simulink model "run_small_function_cov_bf"  (R2022b)
settings: Solver=VariableStepAuto  StartTime=0.0  StopTime=10.0  RelTol=1e-3
libraries: hdlsllib x39, ece1718_small_function x19, simulink x9
settings Model: SimulationMode=accelerator  Creator=kevin  LastModifiedBy=zishu wu

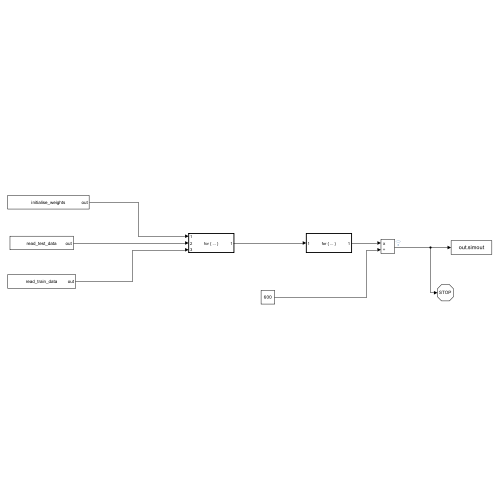
[thumbnail: Simulink's stored preview of the top-level diagram]
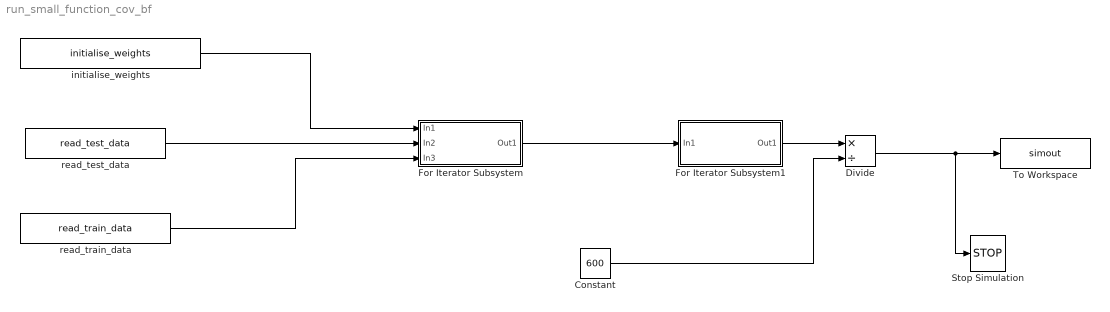
== system run_small_function_cov_bf ==
  Constant : Constant  Value=600
  Divide : Product  Inputs=*/  OutDataTypeStr=double
  For Iterator Subsystem : Subsystem  TreatAsAtomicUnit=on
  For Iterator Subsystem1 : Subsystem  TreatAsAtomicUnit=on
  Stop Simulation : Stop
  To Workspace : ToWorkspace  VariableName=simout  SaveFormat=Timeseries  SampleTime=-1
  initialise_weights : ece1718_small_function/initialise_weights  SampleTime=-1
  read_test_data : ece1718_small_function/read_test_data  SampleTime=-1
  read_train_data : ece1718_small_function/read_train_data  SampleTime=-1
  wires:
  For Iterator Subsystem/1(Out1) -> For Iterator Subsystem1/1(In1)
  read_test_data/1 -> For Iterator Subsystem/2(In2)
  read_train_data/1 -> For Iterator Subsystem/3(In3)
  For Iterator Subsystem1/1(Out1) -> Divide/1
  Constant/1 -> Divide/2
  Divide/1 -> Stop Simulation/1, To Workspace/1
  initialise_weights/1 -> For Iterator Subsystem/1(In1)

== system run_small_function_cov_bf/For Iterator Subsystem ==
  In1 : Inport
  In2 : Inport  Port=2
  In3 : Inport  Port=3
  For Iterator : ForIterator  ResetStates=reset  IterationLimit=1  IndexMode=Zero-based
  train_top : Subsystem  TreatAsAtomicUnit=on
  Out1 : Outport
  wires:
  In1/1 -> Out1/1
  For Iterator/1 -> train_top/1(In1)

== system run_small_function_cov_bf/For Iterator Subsystem1 ==
  In1 : Inport
  Delay : Delay  DelayLength=1  InitialCondition=0
  For Iterator : ForIterator  IterationLimit=600  IndexMode=Zero-based
  validate : ece1718_small_function/validate  SampleTime=-1
  Out1 : Outport
  wires:
  validate/1 -> Delay/1, Out1/1
  For Iterator/1 -> validate/1
  Delay/1 -> validate/2

== system run_small_function_cov_bf/For Iterator Subsystem/train_top ==
  In1 : Inport
  For Iterator : ForIterator  ResetStates=reset  IterationLimit=1  IndexMode=Zero-based
  batch : Subsystem
  Output : Outport
  wires:
  For Iterator/1 -> batch/1(Input)
  In1/1 -> Output/1

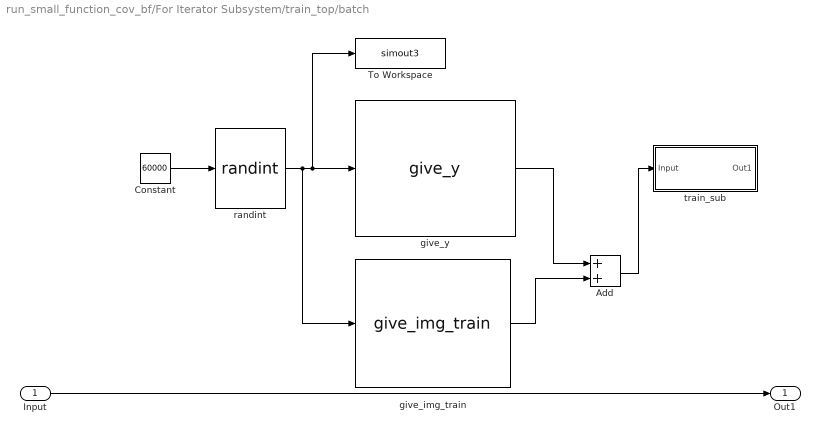
== system run_small_function_cov_bf/For Iterator Subsystem/train_top/batch ==
  Input : Inport
  Add : Sum
  Constant : Constant  Value=60000  OutDataTypeStr=int32
  To Workspace : ToWorkspace  VariableName=simout3  SaveFormat=Timeseries  SampleTime=-1
  give_img_train : ece1718_small_function/give_img_train  SampleTime=-1
  give_y : ece1718_small_function/give_y  SampleTime=-1
  randint : ece1718_small_function/randint  SampleTime=-1
  train_sub : Subsystem
      settings: LibrarySourceBlock=|
      | hdlsllib/Ports &
      | Subsystems/Subsystem
  Out1 : Outport
  wires:
  give_y/1 -> Add/1
  randint/1 -> give_img_train/1, To Workspace/1, give_y/1
  Constant/1 -> randint/1
  Input/1 -> Out1/1
  give_img_train/1 -> Add/2
  Add/1 -> train_sub/1(Input)

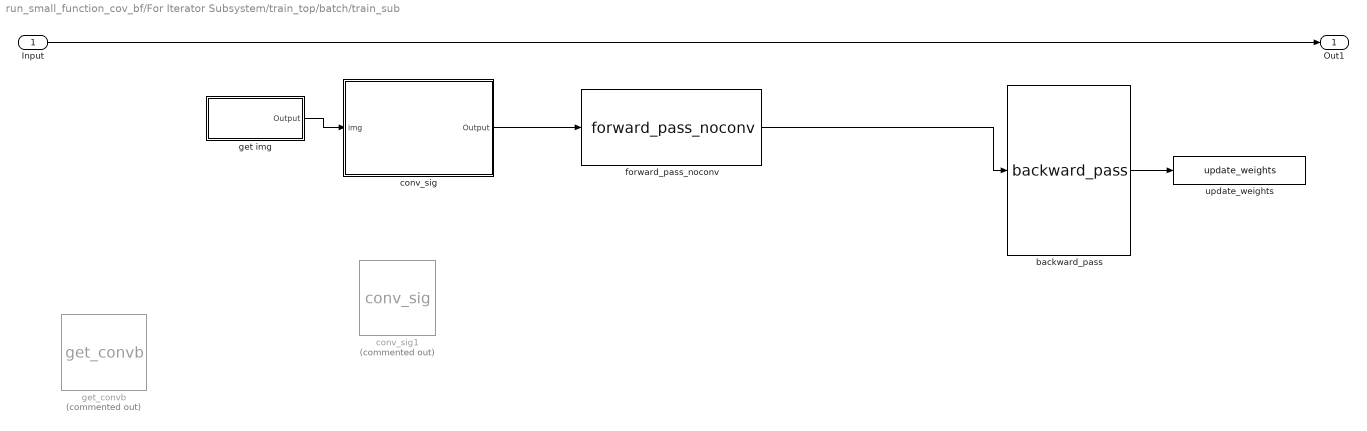
== system run_small_function_cov_bf/For Iterator Subsystem/train_top/batch/train_sub ==
  Input : Inport
  backward_pass : ece1718_small_function/backward_pass  SampleTime=-1
  conv_sig : Subsystem
      settings: LibrarySourceBlock=|
      | hdlsllib/Ports &
      | Subsystems/Subsystem
  conv_sig1 : ece1718_small_function/conv_sig  Commented=on  SampleTime=-1
  forward_pass_noconv : ece1718_small_function/forward_pass_noconv  SampleTime=-1
  get img : Subsystem  TreatAsAtomicUnit=on
  get_convb : ece1718_small_function/get_convb  Commented=on  SampleTime=-1
  update_weights : ece1718_small_function/update_weights  SampleTime=-1
  Out1 : Outport
  wires:
  forward_pass_noconv/1 -> backward_pass/1
  backward_pass/1 -> update_weights/1
  Input/1 -> Out1/1
  get img/1(Output) -> conv_sig/1(img)
  conv_sig/1(Output) -> forward_pass_noconv/1

== system run_small_function_cov_bf/For Iterator Subsystem/train_top/batch/train_sub/conv_sig ==
  img : Inport
  For Iterator : ForIterator  ResetStates=reset  IndexMode=Zero-based
  "filter dim iter " : Subsystem  TreatAsAtomicUnit=on
  filter_ite : ece1718_small_function/filter_ite  Commented=on  SampleTime=-1
  "get_weight " : Subsystem  TreatAsAtomicUnit=on
  Output : Outport
  wires:
  For Iterator/1 -> "get_weight "/1(Input), "filter dim iter "/3(filter_dim)
  img/1 -> "filter dim iter "/1(img)
  "filter dim iter "/1(Output) -> Output/1
  "get_weight "/1(Output) -> "filter dim iter "/2(weight)

== system run_small_function_cov_bf/For Iterator Subsystem/train_top/batch/train_sub/get img ==
  Add : Sum
  Constant : Constant  OutDataTypeStr=int32
  Data Store Memory : DataStoreMemory  WriteAfterWriteMsg=warning  ShowAdditionalParam=off  OutDataTypeStr=uint8  Dimensions=1120
  Data Store Read : DataStoreRead  IndexOptions=Index vector (dialog)  Indices=1  OutputSizes=1
  Data Store Write : DataStoreWrite  EnableIndexing=on  IndexOptions=Index vector (port)  Indices=1  OutputSizes=1
  For Iterator : ForIterator  ResetStates=reset  IterationLimit=1120  IndexMode=Zero-based
  get_img : ece1718_small_function/get_img  SampleTime=-1
  Output : Outport
  wires:
  For Iterator/1 -> Add/2, get_img/1
  get_img/1 -> Data Store Write/1
  Data Store Read/1 -> Output/1
  Constant/1 -> Add/1
  Add/1 -> Data Store Write/2

== system run_small_function_cov_bf/For Iterator Subsystem/train_top/batch/train_sub/conv_sig/filter dim iter  ==
  img : Inport
  weight : Inport  Port=2
  filter_dim : Inport  Port=3
  For Iterator : ForIterator  ResetStates=reset  IterationLimit=28  IndexMode=Zero-based
  i ietar Subsystem : Subsystem  TreatAsAtomicUnit=on
  Output : Outport
  wires:
  img/1 -> i ietar Subsystem/1(img)
  weight/1 -> i ietar Subsystem/2(weight)
  For Iterator/1 -> i ietar Subsystem/3(i)
  filter_dim/1 -> i ietar Subsystem/4(filter_dim)
  i ietar Subsystem/1(Output) -> Output/1

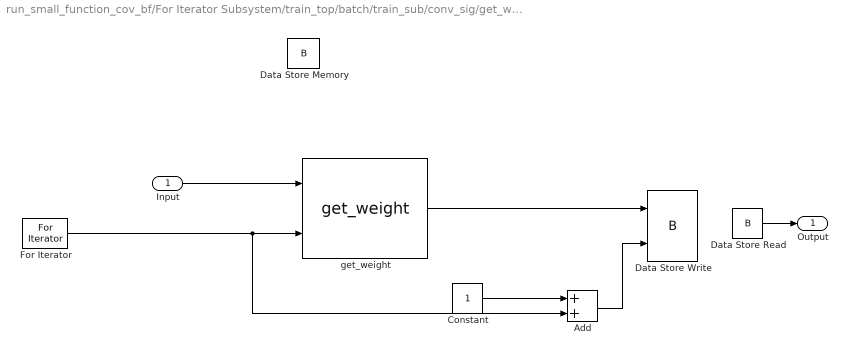
== system run_small_function_cov_bf/For Iterator Subsystem/train_top/batch/train_sub/conv_sig/get_weight  ==
  Input : Inport
  Add : Sum
  Constant : Constant  OutDataTypeStr=int32
  Data Store Memory : DataStoreMemory  DataStoreName=B  ReadBeforeWriteMsg=warning  WriteAfterWriteMsg=warning  ShowAdditionalParam=off  OutDataTypeStr=double  Dimensions=49
  Data Store Read : DataStoreRead  DataStoreName=B  IndexOptions=Index vector (dialog)  Indices=1  OutputSizes=1
  Data Store Write : DataStoreWrite  DataStoreName=B  DataStoreElements=B  EnableIndexing=on  IndexOptions=Index vector (port)  Indices=1  OutputSizes=1
  For Iterator : ForIterator  ResetStates=reset  IterationLimit=49  IndexMode=Zero-based
  get_weight : ece1718_small_function/get_weight  SampleTime=-1
  Output : Outport
  wires:
  For Iterator/1 -> Add/2, get_weight/2
  Input/1 -> get_weight/1
  get_weight/1 -> Data Store Write/1
  Data Store Read/1 -> Output/1
  Constant/1 -> Add/1
  Add/1 -> Data Store Write/2

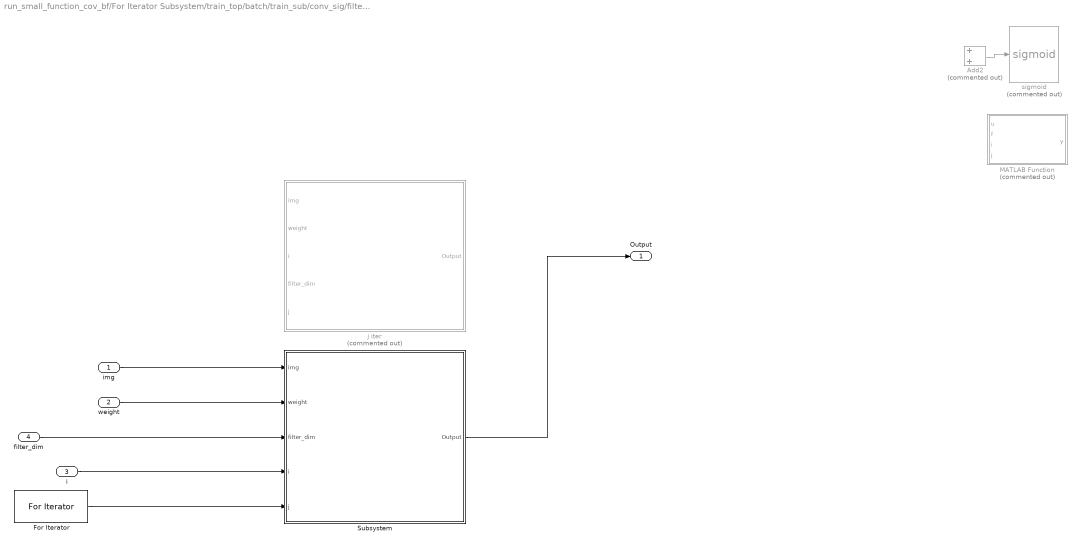
== system run_small_function_cov_bf/For Iterator Subsystem/train_top/batch/train_sub/conv_sig/filter dim iter /i ietar Subsystem ==
  img : Inport
  weight : Inport  Port=2
  i : Inport  Port=3
  filter_dim : Inport  Port=4
  Add2 : Sum  Commented=on
  For Iterator : ForIterator  ResetStates=reset  IterationLimit=28  IndexMode=Zero-based
  MATLAB Function : MATLAB Function  Commented=on  TreatAsAtomicUnit=on
  Subsystem : Subsystem
  j iter : Subsystem  Commented=on
  sigmoid : ece1718_small_function/sigmoid  Commented=on  SampleTime=-1
  Output : Outport
  wires:
  Add2/1 -> sigmoid/1
  For Iterator/1 -> Subsystem/5(j)
  filter_dim/1 -> Subsystem/3(filter_dim)
  i/1 -> Subsystem/4(i)
  weight/1 -> Subsystem/2(weight)
  img/1 -> Subsystem/1(img)
  Subsystem/1(Output) -> Output/1

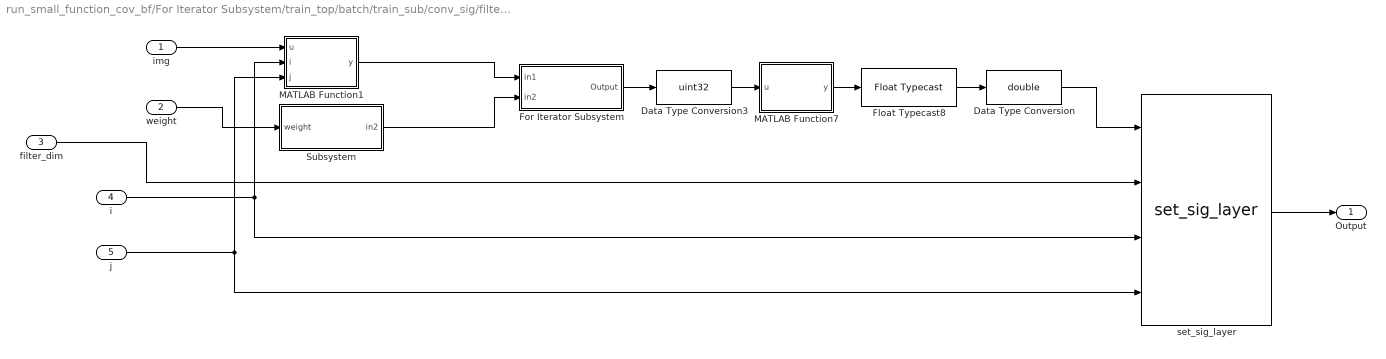
== system run_small_function_cov_bf/For Iterator Subsystem/train_top/batch/train_sub/conv_sig/filter dim iter /i ietar Subsystem/Subsystem ==
  img : Inport
  weight : Inport  Port=2
  filter_dim : Inport  Port=3
  i : Inport  Port=4
  j : Inport  Port=5
  Data Type Conversion : DataTypeConversion  OutDataTypeStr=double  SaturateOnIntegerOverflow=off  RndMeth=Floor
  Data Type Conversion3 : DataTypeConversion  OutDataTypeStr=uint32  SaturateOnIntegerOverflow=off  RndMeth=Floor
  Float Typecast8 : FloatTypecast
  For Iterator Subsystem : Subsystem  TreatAsAtomicUnit=on
  MATLAB Function1 : MATLAB Function  TreatAsAtomicUnit=on
  MATLAB Function7 : MATLAB Function  TreatAsAtomicUnit=on
  Subsystem : Subsystem
  set_sig_layer : ece1718_small_function/set_sig_layer  SampleTime=-1
  Output : Outport
  wires:
  set_sig_layer/1 -> Output/1
  img/1 -> MATLAB Function1/1(u)
  filter_dim/1 -> set_sig_layer/2
  i/1 -> MATLAB Function1/2(i), set_sig_layer/3
  j/1 -> MATLAB Function1/3(j), set_sig_layer/4
  For Iterator Subsystem/1(Output) -> Data Type Conversion3/1
  weight/1 -> Subsystem/1(weight)
  Subsystem/1(in2) -> For Iterator Subsystem/2(in2)
  MATLAB Function1/1(y) -> For Iterator Subsystem/1(in1)
  MATLAB Function7/1(y) -> Float Typecast8/1
  Data Type Conversion3/1 -> MATLAB Function7/1(u)
  Float Typecast8/1 -> Data Type Conversion/1
  Data Type Conversion/1 -> set_sig_layer/1

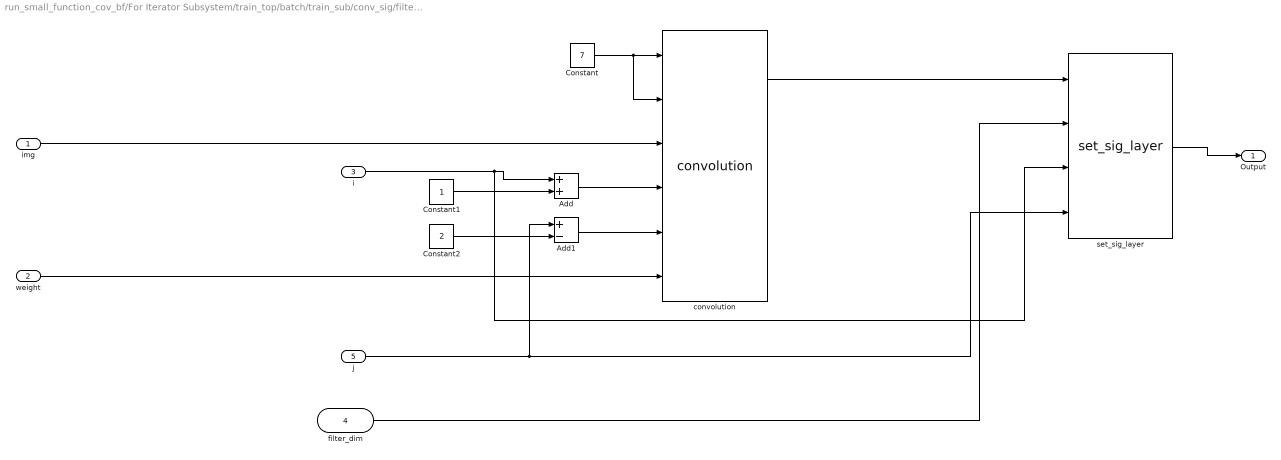
== system run_small_function_cov_bf/For Iterator Subsystem/train_top/batch/train_sub/conv_sig/filter dim iter /i ietar Subsystem/j iter ==
  img : Inport
  weight : Inport  Port=2
  i : Inport  Port=3
  filter_dim : Inport  Port=4
  j : Inport  Port=5
  Add : Sum
  Add1 : Sum  Inputs=+-
  Constant : Constant  Value=7  OutDataTypeStr=int32
  Constant1 : Constant  OutDataTypeStr=int32
  Constant2 : Constant  Value=2  OutDataTypeStr=int32
  convolution : ece1718_small_function/convolution  SampleTime=-1
  set_sig_layer : ece1718_small_function/set_sig_layer  SampleTime=-1
  Output : Outport
  wires:
  Constant2/1 -> Add1/2
  img/1 -> convolution/3
  Constant1/1 -> Add/2
  convolution/1 -> set_sig_layer/1
  Add1/1 -> convolution/5
  Add/1 -> convolution/4
  i/1 -> set_sig_layer/3, Add/1
  filter_dim/1 -> set_sig_layer/2
  Constant/1 -> convolution/2, convolution/1
  weight/1 -> convolution/6
  j/1 -> Add1/1, set_sig_layer/4
  set_sig_layer/1 -> Output/1

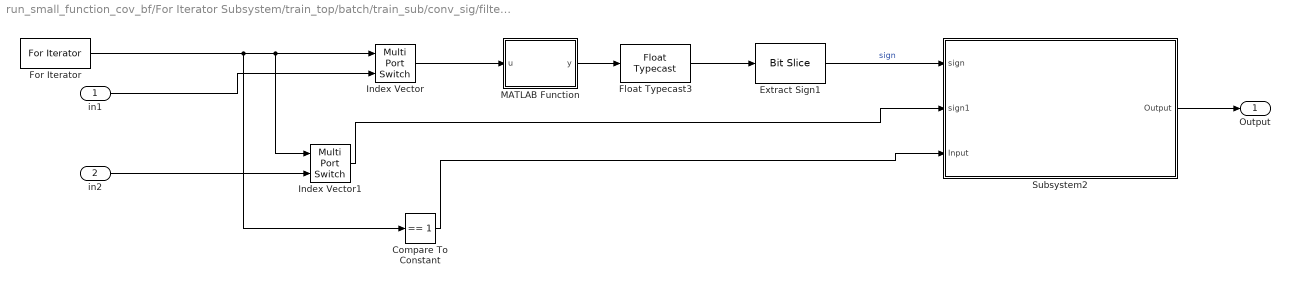
== system run_small_function_cov_bf/For Iterator Subsystem/train_top/batch/train_sub/conv_sig/filter dim iter /i ietar Subsystem/Subsystem/For Iterator Subsystem ==
  in1 : Inport
  in2 : Inport  Port=2
  Compare To Constant : simulink/Logic and Bit Operations/Compare To Constant  relop===  const=1  OutDataTypeStr=boolean
  Extract Sign1 : hdlsllib/Logic and Bit Operations/Bit Slice  lidx=31  ridx=16
  Float Typecast3 : FloatTypecast
  For Iterator : ForIterator  ResetStates=reset  IterationLimit=49
  Index Vector : MultiPortSwitch  Inputs=1  SaturateOnIntegerOverflow=off  InputSameDT=off
  Index Vector1 : MultiPortSwitch  Inputs=1  SaturateOnIntegerOverflow=off  InputSameDT=off
  MATLAB Function : MATLAB Function  TreatAsAtomicUnit=on
  Subsystem2 : Subsystem
  Output : Outport
  wires:
  in1/1 -> Index Vector/2
  in2/1 -> Index Vector1/2
  For Iterator/1 -> Compare To Constant/1, Index Vector1/1, Index Vector/1
  Subsystem2/1(Output) -> Output/1
  Compare To Constant/1 -> Subsystem2/3(Input)
  Index Vector1/1 -> Subsystem2/2(sign1)
  Float Typecast3/1 -> Extract Sign1/1
  MATLAB Function/1(y) -> Float Typecast3/1
  Index Vector/1 -> MATLAB Function/1(u)
  Extract Sign1/1 -> Subsystem2/1(sign)  "sign"

== system run_small_function_cov_bf/For Iterator Subsystem/train_top/batch/train_sub/conv_sig/filter dim iter /i ietar Subsystem/Subsystem/Subsystem ==
  weight : Inport
  Extract Sign1 : hdlsllib/Logic and Bit Operations/Bit Slice  lidx=63  ridx=48
  Float Typecast2 : FloatTypecast
  MATLAB Function : MATLAB Function  TreatAsAtomicUnit=on
  in2 : Outport
  wires:
  weight/1 -> MATLAB Function/1(u)
  MATLAB Function/1(y) -> Float Typecast2/1
  Float Typecast2/1 -> Extract Sign1/1
  Extract Sign1/1 -> in2/1  "sign"

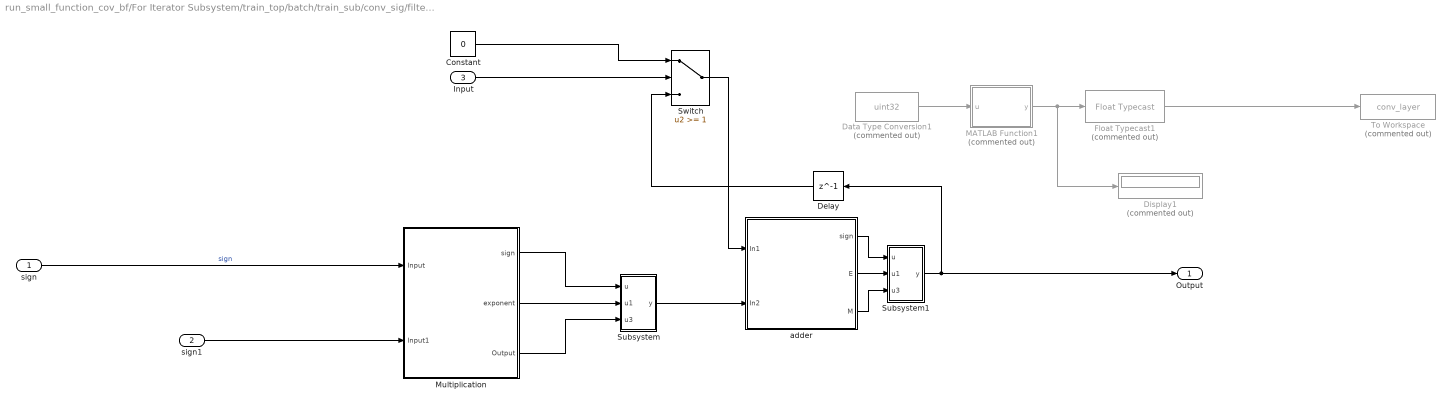
== system run_small_function_cov_bf/For Iterator Subsystem/train_top/batch/train_sub/conv_sig/filter dim iter /i ietar Subsystem/Subsystem/For Iterator Subsystem/Subsystem2 ==
  sign : Inport
  sign1 : Inport  Port=2
  Input : Inport  Port=3
  Constant : Constant  Value=0  OutDataTypeStr=uint16
  Data Type Conversion1 : DataTypeConversion  Commented=on  OutDataTypeStr=uint32  SaturateOnIntegerOverflow=off  RndMeth=Floor
  Delay : Delay  DelayLength=1
  Display1 : Display  Commented=on
  Float Typecast1 : FloatTypecast  Commented=on
  MATLAB Function1 : MATLAB Function  Commented=on  TreatAsAtomicUnit=on
  Multiplication : Subsystem
  Subsystem : Subsystem
  Subsystem1 : Subsystem
  Switch : Switch  Threshold=1  SaturateOnIntegerOverflow=off  InputSameDT=off
  To Workspace : ToWorkspace  Commented=on  VariableName=conv_layer  SaveFormat=Structure With Time  SampleTime=-1
  adder : Subsystem
  Output : Outport
  wires:
  Subsystem1/1(y) -> Output/1, Delay/1
  Delay/1 -> Switch/3
  Input/1 -> Switch/2
  Constant/1 -> Switch/1
  sign1/1 -> Multiplication/2(Input1)
  Multiplication/2(exponent) -> Subsystem/2(u1)
  Multiplication/3(Output) -> Subsystem/3(u3)
  Multiplication/1(sign) -> Subsystem/1(u)
  Subsystem/1(y) -> adder/2(In2)
  sign/1 -> Multiplication/1(Input)  "sign"
  MATLAB Function1/1(y) -> Display1/1, Float Typecast1/1
  Data Type Conversion1/1 -> MATLAB Function1/1(u)
  Float Typecast1/1 -> To Workspace/1
  Switch/1 -> adder/1(In1)
  adder/1(sign) -> Subsystem1/1(u)
  adder/2(E) -> Subsystem1/2(u1)
  adder/3(M) -> Subsystem1/3(u3)

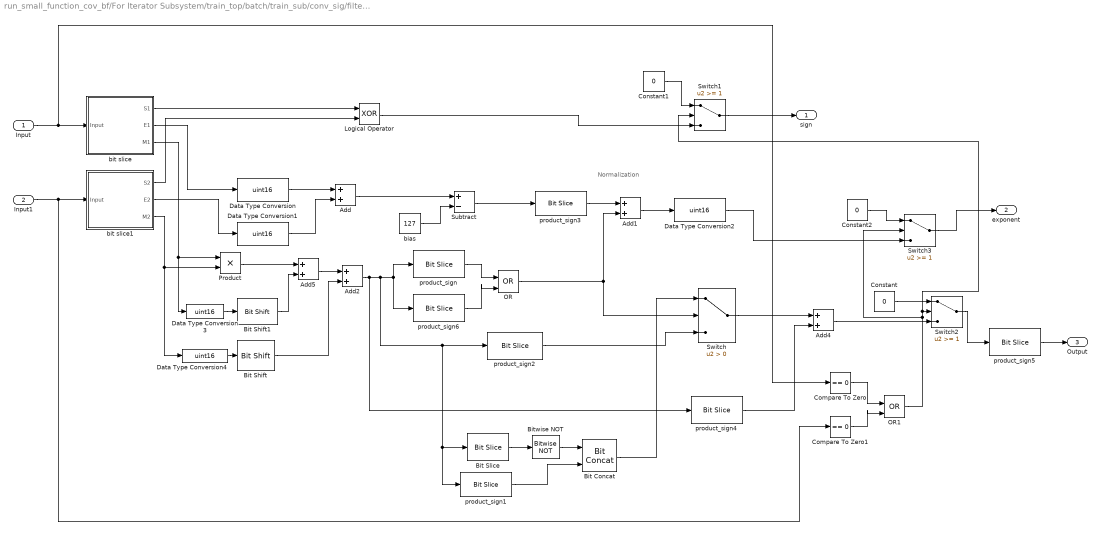
== system run_small_function_cov_bf/For Iterator Subsystem/train_top/batch/train_sub/conv_sig/filter dim iter /i ietar Subsystem/Subsystem/For Iterator Subsystem/Subsystem2/Multiplication ==
  note: Normalization
  Input : Inport
  Input1 : Inport  Port=2
  Add{,2,4..5} (4 alike) : Sum  AccumDataTypeStr=uint16
  Add1 : Sum
  Bit Concat : hdlsllib/Logic and Bit Operations/Bit Concat  numInputs=2
  Bit Shift : hdlsllib/Logic and Bit Operations/Bit Shift  mode=Shift Left Logical  N=7
  Bit Shift1 : hdlsllib/Logic and Bit Operations/Bit Shift  mode=Shift Left Logical  N=7
  Bit Slice : hdlsllib/Logic and Bit Operations/Bit Slice  lidx=14  ridx=14
  Bitwise NOT : simulink/Logic and Bit Operations/Bitwise Operator  logicop=NOT  UseBitMask=off  BitMask=bin2dec('11011001')  BitMaskRealWorld=Stored Integer
      settings: LibrarySourceBlock=|
      | simulink/Quick Insert/Logic and Bit
      | Operations/Bitwise NOT
  Compare To Zero : simulink/Logic and Bit Operations/Compare To Zero  relop===  OutDataTypeStr=boolean
  Compare To Zero1 : simulink/Logic and Bit Operations/Compare To Zero  relop===  OutDataTypeStr=boolean
  Constant : Constant  Value=0  OutDataTypeStr=uint8
  Constant1 : Constant  Value=0  OutDataTypeStr=boolean
  Constant2 : Constant  Value=0  OutDataTypeStr=uint16
  Data Type Conversion{,1..4} (5 alike) : DataTypeConversion  OutDataTypeStr=uint16  SaturateOnIntegerOverflow=off  RndMeth=Floor
  Logical Operator : Logic  Operator=XOR  AllPortsSameDT=off  OutDataTypeStr=boolean
  OR : Logic  Operator=OR  IconShape=distinctive  AllPortsSameDT=off  OutDataTypeStr=boolean
  OR1 : Logic  Operator=OR  IconShape=distinctive  AllPortsSameDT=off  OutDataTypeStr=boolean
  Product : Product  OutDataTypeStr=uint16
  Subtract : Sum  Inputs=+-
  Switch : Switch  Criteria=u2 > Threshold  SaturateOnIntegerOverflow=off  InputSameDT=off
  Switch1 : Switch  Threshold=1  SaturateOnIntegerOverflow=off  InputSameDT=off
  Switch2 : Switch  Threshold=1  SaturateOnIntegerOverflow=off  InputSameDT=off
  Switch3 : Switch  Threshold=1  SaturateOnIntegerOverflow=off  InputSameDT=off
  bias : Constant  Value=127  OutDataTypeStr=uint16
  bit slice : Subsystem
  bit slice1 : Subsystem
  product_sign : hdlsllib/Logic and Bit Operations/Bit Slice  lidx=15  ridx=15
  product_sign1 : hdlsllib/Logic and Bit Operations/Bit Slice  lidx=13  ridx=7
  product_sign2 : hdlsllib/Logic and Bit Operations/Bit Slice  lidx=13  ridx=6
  product_sign3 : hdlsllib/Logic and Bit Operations/Bit Slice  lidx=7  ridx=0
  product_sign4 : hdlsllib/Logic and Bit Operations/Bit Slice  lidx=0  ridx=0
  product_sign5 : hdlsllib/Logic and Bit Operations/Bit Slice  lidx=7  ridx=1
  product_sign6 : hdlsllib/Logic and Bit Operations/Bit Slice  lidx=14  ridx=14
  sign : Outport
  exponent : Outport  Port=2
  Output : Outport  Port=3
  wires:
  Input/1 -> Compare To Zero/1, bit slice/1(Input)
  Input1/1 -> Compare To Zero1/1, bit slice1/1(Input)
  bit slice/1(S1) -> Logical Operator/1
  bit slice1/1(S2) -> Logical Operator/2
  bit slice/2(E1) -> Data Type Conversion/1
  bit slice1/2(E2) -> Data Type Conversion1/1
  Add/1 -> Subtract/1
  Subtract/1 -> product_sign3/1
  bit slice/3(M1) -> Data Type Conversion3/1, Product/1
  bit slice1/3(M2) -> Data Type Conversion4/1, Product/2
  product_sign2/1 -> Switch/3
  Add1/1 -> Data Type Conversion2/1
  product_sign3/1 -> Add1/1
  Add2/1 -> product_sign4/1, product_sign1/1, Bit Slice/1, product_sign2/1, product_sign6/1, product_sign/1
  Data Type Conversion2/1 -> Switch3/3
  Data Type Conversion/1 -> Add/1
  Data Type Conversion1/1 -> Add/2
  bias/1 -> Subtract/2
  Add4/1 -> Switch2/3
  product_sign4/1 -> Add4/2
  Switch/1 -> Add4/1
  Product/1 -> Add5/1
  Add5/1 -> Add2/1
  product_sign5/1 -> Output/1
  Data Type Conversion4/1 -> Bit Shift/1
  Bit Shift/1 -> Add2/2
  Data Type Conversion3/1 -> Bit Shift1/1
  Bit Shift1/1 -> Add5/2
  product_sign/1 -> OR/1
  OR/1 -> Add1/2, Switch/2
  Bit Slice/1 -> Bitwise NOT/1
  Bitwise NOT/1 -> Bit Concat/1
  product_sign1/1 -> Bit Concat/2
  Bit Concat/1 -> Switch/1
  product_sign6/1 -> OR/2
  Switch2/1 -> product_sign5/1
  Compare To Zero/1 -> OR1/1
  Compare To Zero1/1 -> OR1/2
  OR1/1 -> Switch1/2, Switch2/2, Switch3/2
  Constant/1 -> Switch2/1
  Switch1/1 -> sign/1
  Constant1/1 -> Switch1/1
  Logical Operator/1 -> Switch1/3
  Switch3/1 -> exponent/1
  Constant2/1 -> Switch3/1

== system run_small_function_cov_bf/For Iterator Subsystem/train_top/batch/train_sub/conv_sig/filter dim iter /i ietar Subsystem/Subsystem/For Iterator Subsystem/Subsystem2/Subsystem ==
  u : Inport
  u1 : Inport  Port=2
  u3 : Inport  Port=3
  Bit Concat1 : hdlsllib/Logic and Bit Operations/Bit Concat  numInputs=3
  Extract Sign6 : hdlsllib/Logic and Bit Operations/Bit Slice  lidx=7  ridx=0
  Extract Sign7 : hdlsllib/Logic and Bit Operations/Bit Slice  lidx=0  ridx=0
  y : Outport
  wires:
  u/1 -> Extract Sign7/1
  u3/1 -> Bit Concat1/3
  Extract Sign7/1 -> Bit Concat1/1  "sign"
  Extract Sign6/1 -> Bit Concat1/2  "sign"
  u1/1 -> Extract Sign6/1
  Bit Concat1/1 -> y/1

== system run_small_function_cov_bf/For Iterator Subsystem/train_top/batch/train_sub/conv_sig/filter dim iter /i ietar Subsystem/Subsystem/For Iterator Subsystem/Subsystem2/Subsystem1 ==
  u : Inport
  u1 : Inport  Port=2
  u3 : Inport  Port=3
  Bit Concat1 : hdlsllib/Logic and Bit Operations/Bit Concat  numInputs=3
  Extract Sign6 : hdlsllib/Logic and Bit Operations/Bit Slice  lidx=7  ridx=0
  Extract Sign7 : hdlsllib/Logic and Bit Operations/Bit Slice  lidx=0  ridx=0
  y : Outport
  wires:
  u/1 -> Extract Sign7/1
  u3/1 -> Bit Concat1/3
  Extract Sign7/1 -> Bit Concat1/1  "sign"
  Extract Sign6/1 -> Bit Concat1/2  "sign"
  u1/1 -> Extract Sign6/1
  Bit Concat1/1 -> y/1

== system run_small_function_cov_bf/For Iterator Subsystem/train_top/batch/train_sub/conv_sig/filter dim iter /i ietar Subsystem/Subsystem/For Iterator Subsystem/Subsystem2/adder ==
  In1 : Inport
  In2 : Inport  Port=2
  Subsystem3 : Subsystem
  sign : Outport
  E : Outport  Port=2
  M : Outport  Port=3
  wires:
  Subsystem3/1(sign) -> sign/1
  In1/1 -> Subsystem3/1(In1)
  Subsystem3/2(E) -> E/1
  Subsystem3/3(M) -> M/1
  In2/1 -> Subsystem3/2(In2)

== system run_small_function_cov_bf/For Iterator Subsystem/train_top/batch/train_sub/conv_sig/filter dim iter /i ietar Subsystem/Subsystem/For Iterator Subsystem/Subsystem2/Multiplication/bit slice ==
  Input : Inport
  Display : Display
      settings: Format=binary (Stored Integer)
  Extract Exponent : hdlsllib/Logic and Bit Operations/Bit Slice  lidx=14  ridx=7
  Extract Mantissa : hdlsllib/Logic and Bit Operations/Bit Slice  lidx=6  ridx=0
  Extract Sign : hdlsllib/Logic and Bit Operations/Bit Slice  lidx=15  ridx=15
  S1 : Outport
  E1 : Outport  Port=2
  M1 : Outport  Port=3
  wires:
  Input/1 -> Extract Mantissa/1, Extract Exponent/1, Extract Sign/1, Display/1
  Extract Mantissa/1 -> M1/1  "mantissa"
  Extract Sign/1 -> S1/1  "sign"
  Extract Exponent/1 -> E1/1

== system run_small_function_cov_bf/For Iterator Subsystem/train_top/batch/train_sub/conv_sig/filter dim iter /i ietar Subsystem/Subsystem/For Iterator Subsystem/Subsystem2/Multiplication/bit slice1 ==
  Input : Inport
  Extract Exponent : hdlsllib/Logic and Bit Operations/Bit Slice  lidx=14  ridx=7
  Extract Mantissa : hdlsllib/Logic and Bit Operations/Bit Slice  lidx=6  ridx=0
  Extract Sign : hdlsllib/Logic and Bit Operations/Bit Slice  lidx=15  ridx=15
  S2 : Outport
  E2 : Outport  Port=2
  M2 : Outport  Port=3
  wires:
  Input/1 -> Extract Mantissa/1, Extract Exponent/1, Extract Sign/1
  Extract Mantissa/1 -> M2/1  "mantissa"
  Extract Sign/1 -> S2/1  "sign"
  Extract Exponent/1 -> E2/1

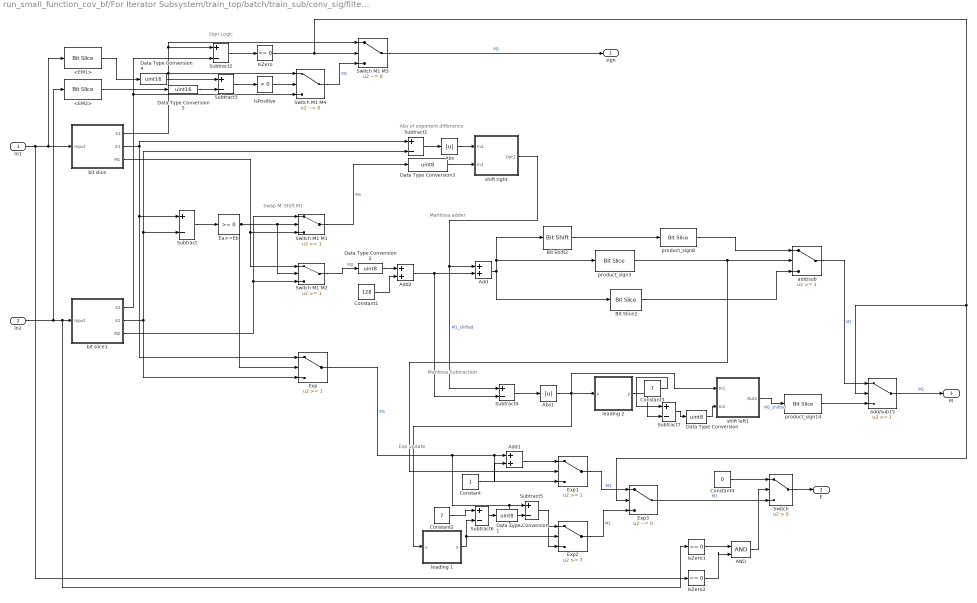
== system run_small_function_cov_bf/For Iterator Subsystem/train_top/batch/train_sub/conv_sig/filter dim iter /i ietar Subsystem/Subsystem/For Iterator Subsystem/Subsystem2/adder/Subsystem3 ==
  note: Mantissa Subtraction
  note: Exp update
  note: Mantissa adder
  note: Sign Logic
  note: Abs of exponent difference
  note: Swap M, Shift M1
  In1 : Inport
  In2 : Inport  Port=2
  <EM1> : hdlsllib/Logic and Bit Operations/Bit Slice  lidx=14  ridx=0
  <EM2> : hdlsllib/Logic and Bit Operations/Bit Slice  lidx=14  ridx=0
  AND : Logic  IconShape=distinctive  AllPortsSameDT=off  OutDataTypeStr=boolean
  Abs : Abs  SaturateOnIntegerOverflow=off
  Abs1 : Abs  SaturateOnIntegerOverflow=off
  Add : Sum  OutDataTypeStr=uint16
  Add1 : Sum
  Add2 : Sum
  Bit Shift2 : hdlsllib/Logic and Bit Operations/Bit Shift  mode=Shift Right Logical  N=1
  Bit Slice2 : hdlsllib/Logic and Bit Operations/Bit Slice  lidx=6  ridx=0
  Constant : Constant  OutDataTypeStr=uint8
  Constant1 : Constant  Value=128  OutDataTypeStr=uint8
  Constant2 : Constant  Value=7
  Constant3 : Constant  Value=7
  Constant4 : Constant  Value=0  OutDataTypeStr=uint8
  Data Type Conversion{,1..3} (4 alike) : DataTypeConversion  OutDataTypeStr=uint8  SaturateOnIntegerOverflow=off  RndMeth=Floor
  Data Type Conversion4 : DataTypeConversion  OutDataTypeStr=uint16  SaturateOnIntegerOverflow=off  RndMeth=Floor
  Data Type Conversion5 : DataTypeConversion  OutDataTypeStr=uint16  SaturateOnIntegerOverflow=off  RndMeth=Floor
  Ea>=Eb : hdlsllib/Logic and Bit Operations/Compare To Zero  relop=>=  OutDataTypeStr=boolean
  Exp : Switch  Threshold=1  SaturateOnIntegerOverflow=off  InputSameDT=off
  Exp1 : Switch  Threshold=1  SaturateOnIntegerOverflow=off  InputSameDT=off
  Exp2 : Switch  Threshold=7  SaturateOnIntegerOverflow=off  InputSameDT=off
  Exp3 : Switch  Criteria=u2 ~= 0  Threshold=1  SaturateOnIntegerOverflow=off  InputSameDT=off
  IsPositive : simulink/Logic and Bit Operations/Compare To Zero  relop=>  OutDataTypeStr=boolean
      settings: LibrarySourceBlock=|
      | simulink/Quick Insert/Logic and Bit
      | Operations/IsPositive
  IsZero : simulink/Logic and Bit Operations/Compare To Zero  relop===  OutDataTypeStr=boolean
      settings: LibrarySourceBlock=|
      | simulink/Quick Insert/Logic and Bit
      | Operations/IsZero
  IsZero1 : simulink/Logic and Bit Operations/Compare To Zero  relop===  OutDataTypeStr=boolean
      settings: LibrarySourceBlock=|
      | simulink/Quick Insert/Logic and Bit
      | Operations/IsZero
  IsZero2 : simulink/Logic and Bit Operations/Compare To Zero  relop===  OutDataTypeStr=boolean
      settings: LibrarySourceBlock=|
      | simulink/Quick Insert/Logic and Bit
      | Operations/IsZero
  Subtract{,1,3..4} (4 alike) : Sum  Inputs=+-  OutDataTypeStr=int16
  Subtract2 : Sum  Inputs=+-  OutDataTypeStr=int8
  Subtract5 : Sum  Inputs=+-  OutDataTypeStr=uint8
  Subtract6 : Sum  Inputs=+-
  Subtract7 : Sum  Inputs=+-
  Switch : Switch  Criteria=u2 > Threshold  SaturateOnIntegerOverflow=off  InputSameDT=off
  Switch M1 M1 : Switch  Threshold=1  SaturateOnIntegerOverflow=off  InputSameDT=off
  Switch M1 M2 : Switch  Threshold=1  SaturateOnIntegerOverflow=off  InputSameDT=off
  Switch M1 M3 : Switch  Criteria=u2 ~= 0  Threshold=1  SaturateOnIntegerOverflow=off  InputSameDT=off
  Switch M1 M4 : Switch  Criteria=u2 ~= 0  Threshold=1  SaturateOnIntegerOverflow=off  InputSameDT=off
  add/sub : Switch  Threshold=1  SaturateOnIntegerOverflow=off  InputSameDT=off
  add/sub15 : Switch  Threshold=1  SaturateOnIntegerOverflow=off  InputSameDT=off
  bit slice : Subsystem
  bit slice1 : Subsystem
  leading 1 : Subsystem
  leading 2 : Subsystem
  product_sign14 : hdlsllib/Logic and Bit Operations/Bit Slice  lidx=6  ridx=0
  product_sign3 : hdlsllib/Logic and Bit Operations/Bit Slice  lidx=8  ridx=8
  product_sign8 : hdlsllib/Logic and Bit Operations/Bit Slice  lidx=6  ridx=0
  shift left1 : Subsystem
  shift right : Subsystem
  sign : Outport
  E : Outport  Port=2
  M : Outport  Port=3
  wires:
  In1/1 -> bit slice/1(Input), <EM1>/1, IsZero2/1
  Subtract/1 -> Ea>=Eb/1
  Ea>=Eb/1 -> Exp/2, Switch M1 M2/2, Switch M1 M1/2
  bit slice/3(M1) -> Switch M1 M1/3, Switch M1 M2/1
  bit slice1/3(M2) -> Switch M1 M2/3, Switch M1 M1/1
  Switch M1 M1/1 -> Data Type Conversion3/1  "M1"
  Subtract1/1 -> Abs/1
  bit slice1/1(S2) -> Switch M1 M4/3, Subtract2/2
  bit slice/1(S1) -> Switch M1 M4/1, Subtract2/1, Switch M1 M3/1
  Subtract2/1 -> IsZero/1
  IsZero/1 -> add/sub15/2, Exp3/2, Switch M1 M3/2
  Abs/1 -> shift right/1(In2)
  shift right/1(Out1) -> Subtract4/1, Add/1  "M1_shifted"
  IsPositive/1 -> Switch M1 M4/2
  Switch M1 M4/1 -> Switch M1 M3/3  "M1"
  Switch M1 M3/1 -> sign/1  "M1"
  Switch M1 M2/1 -> Data Type Conversion2/1  "M2"
  Subtract3/1 -> IsPositive/1
  <EM1>/1 -> Data Type Conversion4/1
  <EM2>/1 -> Data Type Conversion5/1
  Subtract4/1 -> Abs1/1
  Data Type Conversion3/1 -> shift right/2(In1)
  Data Type Conversion2/1 -> Add2/1
  add/sub/1 -> add/sub15/1  "M1"
  Exp/1 -> Exp2/1, Subtract5/1, Add1/1, Exp1/3  "M1"
  product_sign3/1 -> add/sub/2, Exp1/2
  Constant/1 -> Add1/2
  Add1/1 -> Exp1/1
  Subtract5/1 -> Exp2/3
  Add/1 -> Bit Slice2/1, product_sign3/1, Bit Shift2/1
  Bit Shift2/1 -> product_sign8/1
  Bit Slice2/1 -> add/sub/3
  Add2/1 -> Subtract4/2, Add/2
  Constant1/1 -> Add2/2
  product_sign8/1 -> add/sub/1
  product_sign14/1 -> add/sub15/3
  Exp1/1 -> Exp3/1  "M1"
  Exp2/1 -> Exp3/3  "M1"
  Data Type Conversion4/1 -> Subtract3/1
  Data Type Conversion5/1 -> Subtract3/2
  add/sub15/1 -> M/1  "M1"
  leading 1/1(y) -> Exp2/2, Subtract6/2
  Constant2/1 -> Subtract6/1
  leading 2/1(y) -> Subtract7/2
  Constant3/1 -> Subtract7/1
  Abs1/1 -> leading 1/1(u), shift left1/1(In1), leading 2/1(u)
  shift left1/1(Out1) -> product_sign14/1  "M1_shifted"
  bit slice/2(E1) -> Subtract1/1, Subtract/1, Exp/1
  bit slice1/2(E2) -> Exp/3, Subtract/2, Subtract1/2
  Switch/1 -> E/1
  IsZero1/1 -> AND/1
  IsZero2/1 -> AND/2
  AND/1 -> Switch/2
  In2/1 -> bit slice1/1(Input), IsZero1/1, <EM2>/1
  Exp3/1 -> Switch/3  "M1"
  Constant4/1 -> Switch/1
  Subtract7/1 -> Data Type Conversion/1
  Data Type Conversion/1 -> shift left1/2(In2)
  Subtract6/1 -> Data Type Conversion1/1
  Data Type Conversion1/1 -> Subtract5/2

== system run_small_function_cov_bf/For Iterator Subsystem/train_top/batch/train_sub/conv_sig/filter dim iter /i ietar Subsystem/Subsystem/For Iterator Subsystem/Subsystem2/adder/Subsystem3/bit slice ==
  Input : Inport
  Display : Display
      settings: Format=binary (Stored Integer)
  Extract Exponent : hdlsllib/Logic and Bit Operations/Bit Slice  lidx=14  ridx=7
  Extract Mantissa : hdlsllib/Logic and Bit Operations/Bit Slice  lidx=6  ridx=0
  Extract Sign : hdlsllib/Logic and Bit Operations/Bit Slice  lidx=15  ridx=15
  S1 : Outport
  E1 : Outport  Port=2
  M1 : Outport  Port=3
  wires:
  Input/1 -> Extract Mantissa/1, Extract Exponent/1, Extract Sign/1, Display/1
  Extract Mantissa/1 -> M1/1  "mantissa"
  Extract Sign/1 -> S1/1  "sign"
  Extract Exponent/1 -> E1/1

== system run_small_function_cov_bf/For Iterator Subsystem/train_top/batch/train_sub/conv_sig/filter dim iter /i ietar Subsystem/Subsystem/For Iterator Subsystem/Subsystem2/adder/Subsystem3/bit slice1 ==
  Input : Inport
  Display : Display
      settings: Format=binary (Stored Integer)
  Extract Exponent : hdlsllib/Logic and Bit Operations/Bit Slice  lidx=14  ridx=7
  Extract Mantissa : hdlsllib/Logic and Bit Operations/Bit Slice  lidx=6  ridx=0
  Extract Sign : hdlsllib/Logic and Bit Operations/Bit Slice  lidx=15  ridx=15
  S2 : Outport
  E2 : Outport  Port=2
  M2 : Outport  Port=3
  wires:
  Input/1 -> Extract Mantissa/1, Extract Exponent/1, Extract Sign/1, Display/1
  Extract Mantissa/1 -> M2/1  "mantissa"
  Extract Sign/1 -> S2/1  "sign"
  Extract Exponent/1 -> E2/1

== system run_small_function_cov_bf/For Iterator Subsystem/train_top/batch/train_sub/conv_sig/filter dim iter /i ietar Subsystem/Subsystem/For Iterator Subsystem/Subsystem2/adder/Subsystem3/leading 1 ==
  u : Inport
  MATLAB Function : MATLAB Function  TreatAsAtomicUnit=on
  y : Outport
  wires:
  u/1 -> MATLAB Function/1(u)
  MATLAB Function/1(y) -> y/1

== system run_small_function_cov_bf/For Iterator Subsystem/train_top/batch/train_sub/conv_sig/filter dim iter /i ietar Subsystem/Subsystem/For Iterator Subsystem/Subsystem2/adder/Subsystem3/leading 2 ==
  u : Inport
  MATLAB Function : MATLAB Function  TreatAsAtomicUnit=on
  y : Outport
  wires:
  u/1 -> MATLAB Function/1(u)
  MATLAB Function/1(y) -> y/1

== system run_small_function_cov_bf/For Iterator Subsystem/train_top/batch/train_sub/conv_sig/filter dim iter /i ietar Subsystem/Subsystem/For Iterator Subsystem/Subsystem2/adder/Subsystem3/shift left1 ==
  In1 : Inport
  In2 : Inport  Port=2
  Constant : Constant  Value=2  OutDataTypeStr=single
  Data Type Conversion1 : DataTypeConversion  OutDataTypeStr=uint8  SaturateOnIntegerOverflow=off  RndMeth=Floor
  Data Type Conversion2 : DataTypeConversion  OutDataTypeStr=single  SaturateOnIntegerOverflow=off  RndMeth=Floor
  Pow : Math  Operator=pow  SignedPower=on  RndMeth=Zero
  Product : Product
  Out1 : Outport
  wires:
  Pow/1 -> Data Type Conversion1/1
  Constant/1 -> Pow/1
  In2/1 -> Data Type Conversion2/1
  Product/1 -> Out1/1
  Data Type Conversion1/1 -> Product/2
  Data Type Conversion2/1 -> Pow/2
  In1/1 -> Product/1

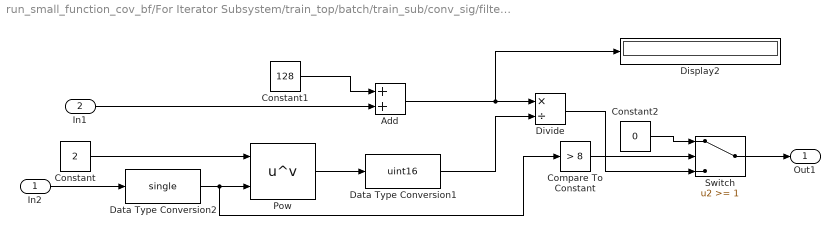
== system run_small_function_cov_bf/For Iterator Subsystem/train_top/batch/train_sub/conv_sig/filter dim iter /i ietar Subsystem/Subsystem/For Iterator Subsystem/Subsystem2/adder/Subsystem3/shift right ==
  In2 : Inport
  In1 : Inport  Port=2
  Add : Sum
  Compare To Constant : simulink/Logic and Bit Operations/Compare To Constant  relop=>  const=8  OutDataTypeStr=boolean
  Constant : Constant  Value=2  OutDataTypeStr=single
  Constant1 : Constant  Value=128  OutDataTypeStr=uint8
  Constant2 : Constant  Value=0  OutDataTypeStr=uint8
  Data Type Conversion1 : DataTypeConversion  OutDataTypeStr=uint16  SaturateOnIntegerOverflow=off  RndMeth=Floor
  Data Type Conversion2 : DataTypeConversion  OutDataTypeStr=single  SaturateOnIntegerOverflow=off  RndMeth=Floor
  Display2 : Display
      settings: Format=binary (Stored Integer)
  Divide : Product  Inputs=*/  RndMeth=Simplest  SaturateOnIntegerOverflow=on
  Pow : Math  Operator=pow  SignedPower=on  RndMeth=Zero
  Switch : Switch  Threshold=1  SaturateOnIntegerOverflow=off  InputSameDT=off
  Out1 : Outport
  wires:
  Pow/1 -> Data Type Conversion1/1
  Constant/1 -> Pow/1
  In2/1 -> Data Type Conversion2/1
  Data Type Conversion1/1 -> Divide/2
  Data Type Conversion2/1 -> Compare To Constant/1, Pow/2
  Add/1 -> Display2/1, Divide/1
  In1/1 -> Add/2
  Constant1/1 -> Add/1
  Compare To Constant/1 -> Switch/2
  Constant2/1 -> Switch/1
  Divide/1 -> Switch/3
  Switch/1 -> Out1/1

== matlab function run_small_function_cov_bf/For Iterator Subsystem/train_top/batch/train_sub/conv_sig/filter dim iter /i ietar Subsystem/MATLAB Function ==
  data: u input; y output; f input; i input; j input
function y = fcn(u,f,i,j)

y = u(f+1,i+1,j+1);
end

== matlab function run_small_function_cov_bf/For Iterator Subsystem/train_top/batch/train_sub/conv_sig/filter dim iter /i ietar Subsystem/Subsystem/MATLAB Function1 ==
  data: u input; y output; i input; j input
function y = img_sampler(u, i, j)
y = zeros([1,49]);
for a = 0:6
    for b = 0:6
        y(a*7+b+1) = u((i+a+1)*32+j+b-2+1); 
    end
end
end

== matlab function run_small_function_cov_bf/For Iterator Subsystem/train_top/batch/train_sub/conv_sig/filter dim iter /i ietar Subsystem/Subsystem/For Iterator Subsystem/Subsystem2/MATLAB Function1 ==
  data: u input; y output
function y = fcn(u)

y = bitshift(u,16);

== matlab function run_small_function_cov_bf/For Iterator Subsystem/train_top/batch/train_sub/conv_sig/filter dim iter /i ietar Subsystem/Subsystem/Subsystem/MATLAB Function ==
  data: u input; y output
function y = fcn(u)
c = CustomFloat(u,16,7);
y = double(c);

== matlab function run_small_function_cov_bf/For Iterator Subsystem/train_top/batch/train_sub/conv_sig/filter dim iter /i ietar Subsystem/Subsystem/MATLAB Function7 ==
  data: u input; y output
function y = fcn(u)

y = bitshift(u,16);

== matlab function run_small_function_cov_bf/For Iterator Subsystem/train_top/batch/train_sub/conv_sig/filter dim iter /i ietar Subsystem/Subsystem/For Iterator Subsystem/MATLAB Function ==
  data: u input; y output
function y = fcn(u)
c = CustomFloat(u,16,7);
y = single(c);

== matlab function run_small_function_cov_bf/For Iterator Subsystem/train_top/batch/train_sub/conv_sig/filter dim iter /i ietar Subsystem/Subsystem/For Iterator Subsystem/Subsystem2/adder/Subsystem3/leading 1/MATLAB Function ==
  data: u input; y output
function y = fcn(u)
v = double(u);
y = floor(log(v)/log(2));

== matlab function run_small_function_cov_bf/For Iterator Subsystem/train_top/batch/train_sub/conv_sig/filter dim iter /i ietar Subsystem/Subsystem/For Iterator Subsystem/Subsystem2/adder/Subsystem3/leading 2/MATLAB Function ==
  data: u input; y output
function y = fcn(u)
v = double(u);
y = floor(log(v)/log(2));
